simulink model "Sensor_Complimantary"  (R2021a)
settings: Solver=FixedStepAuto  StartTime=0.0  StopTime=Inf  RelTol=1e-3  EnableMultiTasking=on
libraries: arduinosensorlib x1
settings Model: SILPILModeSetting=veronly  ExtModeTrigDuration=2  Creator=Samsung  LastModifiedBy=Samsung
settings OptimizationCC: EnhancedBackFolding=on  PassReuseOutputArgsAs=Individual arguments  ZeroExternalMemoryAtStartup=off  ZeroInternalMemoryAtStartup=off  MaxStackSize=64  OptimizeBlockOrder=speed  DifferentSizesBufferReuse=on  OptimizationCustomize=off  EfficientTunableParamExpr=on
settings DebuggingCC: ParameterTunabilityLossMsg=error
settings HardwareCC: ProdBitPerInt=16  ProdBitPerPointer=16  ProdBitPerSizeT=16  ProdBitPerPtrDiffT=16  ProdLargestAtomicFloat=None  ProdWordSize=8  ProdHWDeviceType=Atmel->AVR
settings SFSimCC: MATLABDynamicMemAlloc=off
settings RTWCC: SystemTargetFile=ert.tlc  HardwareBoard=Arduino Uno  TemplateMakefile=ert_default_tmf  Toolchain=Arduino AVR  BuildConfiguration=Faster Runs
settings CodeAppCC: ForceParamTrailComments=on  IgnoreCustomStorageClasses=off  OperatorAnnotations=on  SimulinkDataObjDesc=on  SFDataObjDesc=on  InsertBlockDesc=on
settings ERTTargetCC: SupportContinuousTime=on  SupportVariableSizeSignals=on  ExtModeStaticAllocSize=250

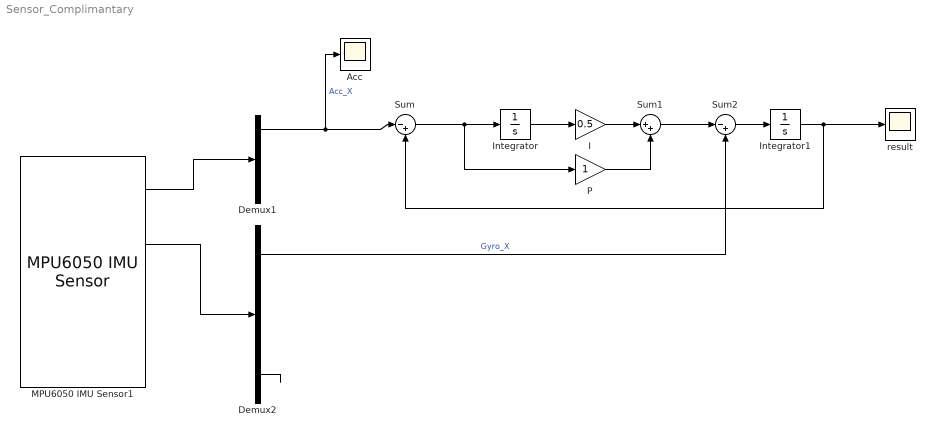
== system Sensor_Complimantary ==
  Acc : Scope
  Demux1 : Demux  Outputs=3
  Demux2 : Demux  Outputs=3
  I : Gain  Gain=0.5
  Integrator : Integrator
  Integrator1 : Integrator
  MPU6050 IMU Sensor1 : arduinosensorlib/MPU6050 IMU Sensor  SlaveAddress=0x68  Accel=on  AngularRate=on  Temperature=on  Status=on  EulerAngles=off  Quat=off  AccelRange=2G  GyroRange=250 dps  DmpOdr=200 Hz  Dlpf=Accelerometer: 184Hz, Gyroscope: 188Hz  SampleTime=-1
      settings: SourceProductBaseCode=ARDUINO
  P : Gain
  Sum : Sum  Inputs=|-+
  Sum1 : Sum  Inputs=|++
  Sum2 : Sum  Inputs=|-+
  result : Scope
  wires:
  Integrator1/1 -> result/1, Sum/2
  Sum2/1 -> Integrator1/1
  P/1 -> Sum1/2
  Demux2/1 -> Sum2/2  "Gyro_X"
  Sum1/1 -> Sum2/1
  I/1 -> Sum1/1
  Integrator/1 -> I/1
  Demux1/1 -> Acc/1, Sum/1  "Acc_X"
  MPU6050 IMU Sensor1/1 -> Demux1/1
  MPU6050 IMU Sensor1/2 -> Demux2/1
  Demux2/3 -> ?
  Sum/1 -> P/1, Integrator/1
